simulink model "Position_control_PP"  (R2019b)
settings: Solver=ode1  StartTime=0.0  StopTime=26  FixedStep=0.002  RelTol=1e-3  EnableMultiTasking=on
PostLoadFcn:
  | qc_set_target_type(getConfigSet(bdroot, 'QUARC Default Target Configuration'));
undefined symbols (not defined in the file): __PRM__SERIALIZED__DATA__, HIL, K0pp, K1pp, qc_get_step_size, SubsystemReferenceBlock
libraries: quarc_library x12, SignalEditorBlockLib x9, simulink_extras x7, cstblocks x7, simulink x2
settings Model: SimulationMode=external  ExtModeTrigDuration=10000  Creator=MLevis  LastModifiedBy=Student
settings SolverCC: PositivePriorityOrder=on
settings DataIOCC: LimitDataPoints=on  SaveFormat=Array  SignalLoggingSaveFormat=ModelDataLogs  ReturnWorkspaceOutputs=off
settings OptimizationCC: ExpressionDepthLimit=2147483647  InitFltsAndDblsToZero=on
settings DebuggingCC: SaveWithParameterizedLinksMsg=none  UnderspecifiedInitializationDetection=Classic  MergeDetectMultiDrivingBlocksExec=none  SolverPrmCheckMsg=warning  MultiTaskDSMMsg=warning  MultiTaskCondExecSysMsg=none  FcnCallInpInsideContextMsg=warning  StateNameClashWarn=warning  SFUnexpectedBacktrackingDiag=warning  SFNoUnconditionalDefaultTransitionDiag=warning  SFExecutionAtInitializationDiag=none  ArithmeticOperatorsInVariantConditions=warning
settings HardwareCC: ProdBitPerPointer=32  ProdBitPerSizeT=32  ProdBitPerPtrDiffT=32  ProdLargestAtomicFloat=None  ProdIntDivRoundTo=Undefined  ProdEndianess=Unspecified  ProdWordSize=32  ProdHWDeviceType=32-bit Generic
settings ModelReferenceCC: PropagateSignalLabelsOutOfModel=off
settings SFSimCC: SimUseLocalCustomCode=off  CustomCodeUndefinedFunction=UseInterfaceOnly
settings RTWCC: Description=QUARC Win64 Target  SystemTargetFile=quarc_win64.tlc  TemplateMakefile=quarc_default_tmf  RTWUseLocalCustomCode=off
settings CodeAppCC: StateflowObjectComments=on
settings STFCustomTargetCC: TargetPreCompLibLocation=C:\PROGRA~3\QUARC\lib\2019b\win64\release  ConcurrentExecutionCompliant=on  GRTInterface=on  SystemTargetFile=quarc_win64.tlc
settings GRTTargetCC: TargetPreCompLibLocation=C:\PROGRA~3\QUARC\lib\2019b\win64\release  TargetLangStandard=C89/C90 (ANSI)  ParMdlRefBuildCompliant=off  CompOptLevelCompliant=off  CombineOutputUpdateFcns=off  MatFileLogging=off  CPPClassGenCompliant=off  GRTInterface=on  UseToolchainInfoCompliant=off  ExtMode=on  ExtModeMexFile=quarc_comm
settings ConfigComp: CovMetricSettings=dw  CovHtmlReporting=on  CovSaveCumulativeToWorkspaceVar=on  CovSaveSingleToWorkspaceVar=on  CovExternalEMLEnable=off

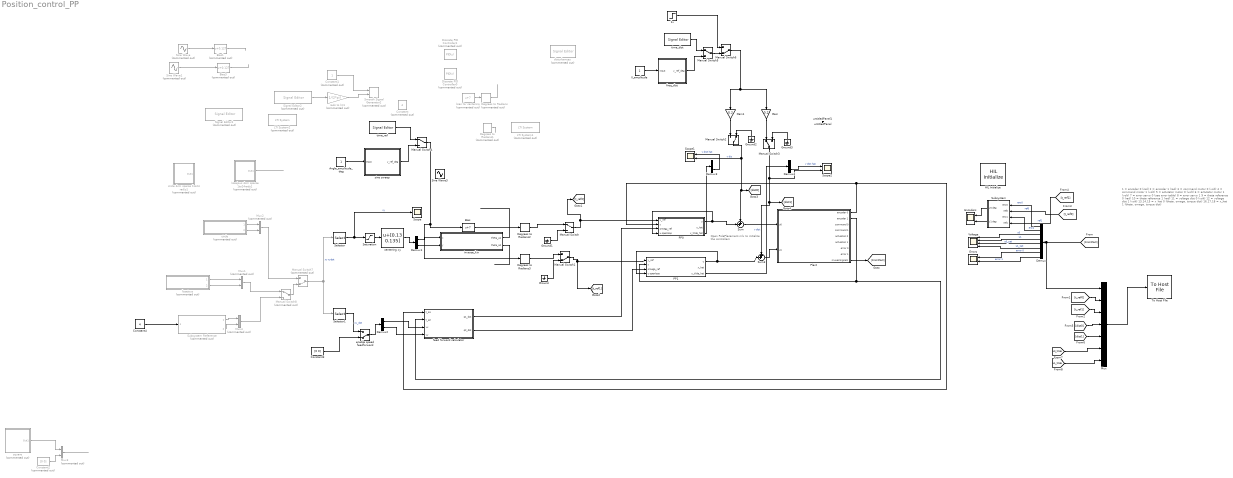
== system Position_control_PP ==
  note: Open PolePlacement.mlx
      | to initialize the controllers
  note: 1 = encoder 0 (rad)
      | 2 = encoder 1 (rad)
      | 3 = command motor 0 (volt)
      | 4 = command motor 1 (volt)
      | 5 = actutator motor 0 (volt)
      | 6 = actutator motor 1 (volt)
      | 7 = error servo 0 (see error table)
      | 8 = error servo 1
      | 9 = theta reference 0 (rad)
      | 10 = theta reference 1 (rad)
      | 11 = voltage dist 0 (volt)
      | 12 = voltage dist 1 (volt)
      | 13,14,15 = x_hat 0 (theta, omega, torque dist)
      | 16,17,18 = x_hat 1 (theta, omega, torque dist)
  1v : Step  SampleTime=0
  Angle_amplitude_deg : Constant
  Bias : Bias  Bias=7
  Bias1 : Bias  Commented=on  Bias=0.127
  Bias3 : Bias  Commented=on  Bias=0.127
  Constant : Constant  Commented=on  Value=4
  Constant1 : Constant  Commented=on
  Constant2 : Constant  Commented=on  Value=[0 0]
  Constant3 : Constant  Value=[0 0]
  Constant4 : Constant  Value=4
  Degrees to Radians : simulink_extras/Transformations/Degrees to Radians  Commented=on
  Degrees to Radians1 : simulink_extras/Transformations/Degrees to Radians  Commented=on
  Degrees to Radians2 : simulink_extras/Transformations/Degrees to Radians
  Degrees to Radians3 : simulink_extras/Transformations/Degrees to Radians
  Demux : Demux  Outputs=8
  Demux1 : Demux  Outputs=2
  Demux2 : Demux  Outputs=2
  Demux3 : Demux  Outputs=3
  Demux4 : Demux  Outputs=3
  Discrete PID Controller0 : simulink/Continuous/PID Controller  Commented=on  Controller=PID  Form=Parallel  TimeDomain=Discrete-time  SampleTime=-1  IntegratorMethod=Forward Euler  FilterMethod=Forward Euler  ControllerParametersSource=internal  P=-21.6  I=0  D=-0.423  UseFilter=on  N=100  TunerSelectOption=Transfer Function Based (PID Tuner App)  InitialConditionSource=internal  InitialConditionForIntegrator=0  InitialConditionForFilter=0  DifferentiatorICPrevScaledInput=0  ExternalReset=none  TrackingMode=off  Kt=1  LimitOutput=off  UpperSaturationLimit=inf  LowerSaturationLimit=-inf  LinearizeAsGain=off  AntiWindupMode=none  Kb=1  POutMin=[]  POutMax=[]  IOutMin=[]  IOutMax=[]  DOutMin=[]  DOutMax=[]  NOutMin=[]  NOutMax=[]  SumOutMin=[]  SumOutMax=[]  SaturationOutMin=[]  SaturationOutMax=[]  PParamMin=[]  PParamMax=[]  IParamMin=[]  IParamMax=[]  DParamMin=[]  DParamMax=[]  NParamMin=[]  NParamMax=[]  KbParamMin=[]  KbParamMax=[]  KtParamMin=[]  KtParamMax=[]  KbOutMin=[]  KbOutMax=[]  KtOutMin=[]  KtOutMax=[]  IntegratorOutMin=[]  IntegratorOutMax=[]  FilterOutMin=[]  FilterOutMax=[]  SumI1OutMin=[]  SumI1OutMax=[]  SumI2OutMin=[]  SumI2OutMax=[]  SumI3OutMin=[]  SumI3OutMax=[]  SumI4OutMin=[]  SumI4OutMax=[]  SumDOutMin=[]  SumDOutMax=[]  DifferentiatorOutMin=[]  DifferentiatorOutMax=[]  FilterDiffOutCoefMin=[]  FilterDiffOutCoefMax=[]  ReciprocalOutMin=[]  ReciprocalOutMax=[]  SumDenOutMin=[]  SumDenOutMax=[]  SumNumOutMin=[]  SumNumOutMax=[]  DivideOutMin=[]  DivideOutMax=[]  IntegratorContinuousStateAttributes=''  IntegratorStateMustResolveToSignalObject=off  IntegratorRTWStateStorageClass=Auto  FilterContinuousStateAttributes=''  FilterStateMustResolveToSignalObject=off  FilterRTWStateStorageClass=Auto  ParallelPVariant=InternalParameters  IdealPVariant=Disabled  IVariant=InternalParameters  DVariant=InternalParameters  IntegratorVariant=Discrete  SatVariant=Disabled  AWVariant=Passthrough  PCopyVariant=Disabled  TRVariant=Disabled  FdbkBlocksVariant=Forward  IdealPFdbkVariant=Disabled  SatFdbkVariant=Disabled  DerivativeFilterVariant=ForwardEulerFilter  NVariant=InternalParameters  NCopyVariant=Disabled  FilterICVariant=InternalICsFilter  IntegratorICVariant=InternalICs  ExternalResetVariant=Disabled  TRSumVariant=Passthrough  SumFdbkVariant=Disabled  SumVariant=Sum_PID
  Discrete PID Controller1 : simulink/Continuous/PID Controller  Commented=on  Controller=PID  Form=Parallel  TimeDomain=Discrete-time  SampleTime=-1  IntegratorMethod=Forward Euler  FilterMethod=Forward Euler  ControllerParametersSource=internal  P=-21.4  I=0  D=-0.43  UseFilter=on  N=100  TunerSelectOption=Transfer Function Based (PID Tuner App)  InitialConditionSource=internal  InitialConditionForIntegrator=0  InitialConditionForFilter=0  DifferentiatorICPrevScaledInput=0  ExternalReset=none  TrackingMode=off  Kt=1  LimitOutput=off  UpperSaturationLimit=inf  LowerSaturationLimit=-inf  LinearizeAsGain=off  AntiWindupMode=none  Kb=1  POutMin=[]  POutMax=[]  IOutMin=[]  IOutMax=[]  DOutMin=[]  DOutMax=[]  NOutMin=[]  NOutMax=[]  SumOutMin=[]  SumOutMax=[]  SaturationOutMin=[]  SaturationOutMax=[]  PParamMin=[]  PParamMax=[]  IParamMin=[]  IParamMax=[]  DParamMin=[]  DParamMax=[]  NParamMin=[]  NParamMax=[]  KbParamMin=[]  KbParamMax=[]  KtParamMin=[]  KtParamMax=[]  KbOutMin=[]  KbOutMax=[]  KtOutMin=[]  KtOutMax=[]  IntegratorOutMin=[]  IntegratorOutMax=[]  FilterOutMin=[]  FilterOutMax=[]  SumI1OutMin=[]  SumI1OutMax=[]  SumI2OutMin=[]  SumI2OutMax=[]  SumI3OutMin=[]  SumI3OutMax=[]  SumI4OutMin=[]  SumI4OutMax=[]  SumDOutMin=[]  SumDOutMax=[]  DifferentiatorOutMin=[]  DifferentiatorOutMax=[]  FilterDiffOutCoefMin=[]  FilterDiffOutCoefMax=[]  ReciprocalOutMin=[]  ReciprocalOutMax=[]  SumDenOutMin=[]  SumDenOutMax=[]  SumNumOutMin=[]  SumNumOutMax=[]  DivideOutMin=[]  DivideOutMax=[]  IntegratorContinuousStateAttributes=''  IntegratorStateMustResolveToSignalObject=off  IntegratorRTWStateStorageClass=Auto  FilterContinuousStateAttributes=''  FilterStateMustResolveToSignalObject=off  FilterRTWStateStorageClass=Auto  ParallelPVariant=InternalParameters  IdealPVariant=Disabled  IVariant=InternalParameters  DVariant=InternalParameters  IntegratorVariant=Discrete  SatVariant=Disabled  AWVariant=Passthrough  PCopyVariant=Disabled  TRVariant=Disabled  FdbkBlocksVariant=Forward  IdealPFdbkVariant=Disabled  SatFdbkVariant=Disabled  DerivativeFilterVariant=ForwardEulerFilter  NVariant=InternalParameters  NCopyVariant=Disabled  FilterICVariant=InternalICsFilter  IntegratorICVariant=InternalICs  ExternalResetVariant=Disabled  TRSumVariant=Passthrough  SumFdbkVariant=Disabled  SumVariant=Sum_PID
  Encoders : Scope  NumInputPorts=2
  Errors : Scope  NumInputPorts=2
  Gain : Gain  Gain=0.2
  Gain1 : Gain  Gain=0.2
  Ground{,1..3} (4 alike) : Ground
  HIL Initialize : quarc_library/Data Acquisition/Generic/Configuration/HIL Initialize  object_name=HIL-1  board_type=q2_usb  board_number=0  board_options=d0=digital;d1=digital;led=auto;update_rate=normal;decimation=1  exclusive=off  active=off  hardware_clocks=[0]  clock_modes=[]  initial_clock_frequencies=[]  set_clock_params_at_start=off  set_clock_params_at_switch_in=off  set_clock_frequencies_at_start=off  set_clock_frequencies_at_switch_in=off  analog_input_channels=[0:1]  analog_input_configurations=[]  analog_input_maximums=10  analog_input_minimums=-10  set_analog_input_params_at_start=on  set_analog_input_params_at_switch_in=off  analog_output_channels=[0:1]  analog_output_maximums=10  analog_output_minimums=-10  initial_analog_outputs=[0]  final_analog_outputs=[0]  watchdog_analog_outputs=0  set_analog_output_params_at_start=on  set_analog_output_params_at_switch_in=off  set_analog_outputs_at_start=on  set_analog_outputs_at_switch_in=off  set_analog_outputs_at_terminate=on  set_analog_outputs_at_switch_out=off  set_analog_outputs_on_watchdog=off  digital_input_channels=[]  digital_output_channels=[]  digital_output_configuration=[]  initial_digital_outputs=[1]  final_digital_outputs=[1]  watchdog_digital_outputs=[1]  set_digital_output_params_at_start=off  set_digital_output_params_at_switch_in=off  set_digital_outputs_at_start=on  set_digital_outputs_at_switch_in=off  set_digital_outputs_at_terminate=on  set_digital_outputs_at_switch_out=off  set_digital_outputs_on_watchdog=off  encoder_channels=[0:1]  quadrature=[4]  encoder_filter_frequency=[]  initial_encoder_counts=[0]  set_encoder_params_at_start=on  set_encoder_params_at_switch_in=off  set_encoder_counts_at_start=on  set_encoder_counts_at_switch_in=off  pwm_channels=[]  pwm_modes=[0]  pwm_frequency=1/0.020  pwm_configuration=[]  pwm_alignment=[]  pwm_polarity=[]  pwm_leading_deadband=[]  pwm_trailing_deadband=[]  initial_pwm_outputs=[0]  final_pwm_outputs=[0]  watchdog_pwm_outputs=[0]  set_pwm_params_at_start=on  set_pwm_params_at_switch_in=off  set_pwm_outputs_at_start=on  set_pwm_outputs_at_switch_in=off  set_pwm_outputs_at_terminate=on  set_pwm_outputs_at_switch_out=off  set_pwm_outputs_on_watchdog=off  other_output_channels=[]  initial_other_outputs=[]  final_other_outputs=[]  watchdog_other_outputs=[]  set_other_outputs_at_start=off  set_other_outputs_at_switch_in=off  set_other_outputs_at_terminate=off  set_other_outputs_at_switch_out=off  set_other_outputs_on_watchdog=off
  LTI System1 : cstblocks/LTI System  Commented=on  sys=C1  IC=[]
  LTI System2 : cstblocks/LTI System  Commented=on  sys=C0  IC=[]
  Manual Switch{,3..5} (4 alike) : ManualSwitch
  Manual Switch1 : ManualSwitch  CurrentSetting=0
  Manual Switch2 : ManualSwitch  CurrentSetting=0
  Manual Switch6 : ManualSwitch  CurrentSetting=0
  Manual Switch7 : ManualSwitch  Commented=on  CurrentSetting=0
  Manual Switch8 : ManualSwitch  Commented=on
  Mux : Mux  Inputs=7
  Mux{1..4} (4 alike) : Mux  Commented=on  Inputs=2
  PP0 : Subsystem
  PP1 : Subsystem
  Plant : Subsystem  mask(Plant with checks){LowSat=10.0, HighSat=0.330, A0min=-17, A0max=31, A0slack=1, bias=off, A1min=-27, A1max=27, A1slack=1}
      mask prompts: LowSat "Nominal Saturation"; HighSat "Safety Saturation"; A0min "A1 Min"; A0max "A1 Max"; A0slack "A1 Slack"; bias "Use cartesian reference"; A1min "A2 Min"; A1max "A2 Max"; A1slack "A2 Slack"
      mask help: All angles described in DEGREES with respect to the markings on the physical system (unless the toggle is checked)
      mask DialogControl Container9 Prompt: Voltages
      mask DialogControl Container9_copy Prompt: Angle Limits
      mask DialogControl ParameterGroupVar Prompt: Theta A1 (Motor 0)
      mask DialogControl Container8 Prompt: Theta A2 (Motor 1)
      mask DialogControl Control2 Prompt: When enabled uses the canonical angles instead of the displacement from resting position
      mask Display: image('$imagefile'); % Use "Edit Image" on toolstrip to change.
  Saturation : Saturate  UpperLimit=0.04  LowerLimit=-0.04
  Scope : Scope
  Scope1 : Scope  NumInputPorts=2
  Scope2 : Scope  NumInputPorts=2
  Selector : Selector  InputPortWidth=4  IndexOptions=Index vector (dialog)  Indices=[1 2]  OutputSizes=1
  Selector1 : Selector  InputPortWidth=4  IndexOptions=Index vector (dialog)  Indices=[3 4]  OutputSizes=1
  Signal Editor1 : SignalEditorBlockLib/Signal Editor  Commented=on  FileName=D:\Users\icpmoles\my\polimi\università\Magistrale 2 anno 2 semestre\lab\ASB\lab5\preplan\stairs.mat  ActiveScenario=x1to35sparse  ActiveSignal=Signal  IsBus=off  OutputBusObjectStr=Bus: BusObject  SampleTime=0  Interpolate=off  ZeroCross=off  OutputAfterFinalValue=Setting to zero  Unit=inherit  PreserveSignalName=on
      settings: SourceProductName=Simulink
  Signal Editor2 : SignalEditorBlockLib/Signal Editor  Commented=on  FileName=C:\Users\Student\Downloads\CNC (4)\CNC\sinesweep\lab4\stairs.mat  ActiveScenario=x1to30with10s_pause  ActiveSignal=Signal 1  IsBus=off  OutputBusObjectStr=Bus: BusObject  SampleTime=0  Interpolate=off  ZeroCross=off  OutputAfterFinalValue=Holding final value  Unit=inherit  PreserveSignalName=on
      settings: SourceProductName=Simulink
  Sine Wave : Sin  Commented=on  Amplitude=0.03  Frequency=2  Phase=pi/2  SampleTime=0
  Sine Wave1 : Sin  Commented=on  Amplitude=0.03  Frequency=2  SampleTime=0
  Sine Wave3 : Sin  Amplitude=0.5  Frequency=5  SampleTime=0
  Smooth Signal Generator2 : quarc_library/Sources/Signals/Smooth Signal Generator  Commented=on  signal_type=Sine  source=External (input ports)  amplitude=1  frequency=1  initial_phase=0  sample_time=qc_get_step_size  output_cos=off
      settings: SourceProductName=QUARC Targets
  Subsystem : Subsystem
  Subsystem Reference : Subsystem  Commented=on  BlockKeywords=__PRM__SERIALIZED__DATA__:SubsystemReferenceBlock  ReferencedSubsystem=square_generator
  Sum : Sum  Inputs=++|
  Sum3 : Sum  Inputs=++|
  To Host File : quarc_library/Sinks/To Host/To Host File  file_name=%m_%{date}_%{time}.mat  variable_name=data  decimation=1  sample_time=-1  file_format=MAT-file v.4  options=No header or footer  append=off  final_file_name=Position_control_PP_29-Apr-2025_18-49-00.mat  bitrate=2000000
  V_amplitude : Constant
  Voltage : Scope  NumInputPorts=4
  bias for centering : Bias  Commented=on  Bias=7
  centering xy : Bias  Bias=[0.13 0.135]
  circle : Subsystem  Commented=on  BlockKeywords=__PRM__SERIALIZED__DATA__:SubsystemReferenceBlock  ReferencedSubsystem=circle_generator
  circle 4cm sparse 1to24 rad/s1 : Subsystem  Commented=on
  disturbances : SignalEditorBlockLib/Signal Editor  Commented=on  FileName=D:\Users\icpmoles\my\polimi\università\Magistrale 2 anno 2 semestre\lab\ASB\lab5\preplan\scenario.mat  ActiveScenario=WhiteNoise  ActiveSignal=m0  IsBus=off  OutputBusObjectStr=Bus: BusObject  SampleTime=0  Interpolate=off  ZeroCross=off  OutputAfterFinalValue=Setting to zero  Unit=V  PreserveSignalName=on
      settings: SourceProductName=Simulink
  enable speed feedforward : ManualSwitch  CurrentSetting=0
  feed forward calculator : MATLAB Function  TreatAsAtomicUnit=on
  freq_dist : Subsystem
  "inverse_kin " : Subsystem
  lissajous : Subsystem  Commented=on  BlockKeywords=__PRM__SERIALIZED__DATA__:SubsystemReferenceBlock  ReferencedSubsystem=lissajous_generator
  lissajous 4cm sparse 1to24rads1 : Subsystem  Commented=on
  rads to hz1 : Gain  Commented=on  Gain=1/(2*pi)
  sine sweep : Subsystem
  square : Subsystem  Commented=on
  time_dist : SignalEditorBlockLib/Signal Editor  FileName=angle_ref_scenario_time.mat  ActiveScenario=whitenoise_5to1  ActiveSignal=Signal  IsBus=off  OutputBusObjectStr=Bus: BusObject  SampleTime=0  Interpolate=off  ZeroCross=off  OutputAfterFinalValue=Setting to zero  Unit=inherit  PreserveSignalName=on
      settings: SourceProductName=Simulink
  time_ref : SignalEditorBlockLib/Signal Editor  FileName=angle_ref_scenario_time.mat  ActiveScenario=square_dyn_15to5  ActiveSignal=Signal  IsBus=off  OutputBusObjectStr=Bus: BusObject  SampleTime=0  Interpolate=off  ZeroCross=off  OutputAfterFinalValue=Setting to zero  Unit=inherit  PreserveSignalName=on
      settings: SourceProductName=Simulink
  untitledPanel : Subsystem  Tag=HiddenForWebPanel  IsWebBlockPanel=on
  untitledPanel1 : Subsystem  Tag=HiddenForWebPanel  IsWebBlockPanel=on
  wires:
  Plant/1(encoder 0) -> PP0/2(y), feed forward calculator/1(t_a1)
  Plant/2(encoder 1) -> PP1/2(y), feed forward calculator/2(t_a2)
  PP0/1(u) -> PP0/4(u openloop), Sum/2
  Plant/9(muxed signals) -> [FromPlant]
  [FromPlant] -> Mux/1, Demux/1
  Demux/2 -> Subsystem/3(enc1)  "enc1"
  Demux/3 -> Voltage/1  "u0"
  Demux/4 -> Voltage/2  "u1"
  Demux/5 -> Voltage/3  "u0_sat"
  Demux/6 -> Voltage/4  "u1_sat"
  Demux/7 -> Errors/1  "error 0"
  Demux/8 -> Errors/2  "error 1"
  Manual Switch1/1 -> PP1/1(y_ref), [t_ref1]
  Sum/1 -> Plant/1(u0)
  PP1/1(u) -> PP1/4(u openloop), Sum3/2
  Sum3/1 -> Plant/2(u1)
  Mux/1 -> To Host File/1
  Manual Switch/1 -> [t_ref0], PP0/1(y_ref)
  [t_ref0] -> Mux/2
  [t_ref1] -> Mux/3
  Degrees to Radians/1 -> ?
  Degrees to Radians1/1 -> ?
  Ground/1 -> Manual Switch1/2
  Ground1/1 -> Manual Switch/2
  Manual Switch2/1 -> [dist0], Sum/1, Scope1/2  "v dis"
  Ground2/1 -> Manual Switch2/2
  bias for centering/1 -> Degrees to Radians/1
  Gain/1 -> Manual Switch3/1
  Gain1/1 -> Manual Switch2/1
  [dist0] -> Mux/4
  [dist1] -> Mux/5
  rads to hz1/1 -> Smooth Signal Generator2/2
  Constant1/1 -> Smooth Signal Generator2/1
  Signal Editor2/1 -> rads to hz1/1
  Bias1/1 -> ?
  Bias3/1 -> ?
  Sine Wave/1 -> Bias1/1
  Sine Wave1/1 -> Bias3/1
  Ground3/1 -> Manual Switch3/2
  [t_ref0] -> Subsystem/2(ref0)  "ref0"
  Demux/1 -> Subsystem/1(enc0)  "enc0"
  [t_ref1] -> Subsystem/4(ref1)  "ref1"
  Subsystem/1(y0 deg) -> Encoders/1
  Subsystem/2(y1 deg) -> Encoders/2
  ? -> Degrees to Radians1/1, bias for centering/1
  time_ref/1 -> Manual Switch4/1
  time_dist/1 -> Manual Switch5/1
  freq_dist/1(y_ref_deg) -> Manual Switch5/2
  Manual Switch6/1 -> Gain/1, Gain1/1
  V_amplitude/1 -> freq_dist/1(Input)
  Angle_amplitude_deg/1 -> sine sweep/1(Input)
  [x0_tilde] -> Mux/6
  [x1_tilde] -> Mux/7
  Manual Switch4/1 -> Bias/1, Degrees to Radians3/1
  lissajous 4cm sparse 1to24rads1/1(Out1) -> ?
  Mux2/1 -> Manual Switch7/1
  Manual Switch7/1 -> Selector1/1, Selector/1  "xy xydot"
  Demux1/1 -> "inverse_kin "/1(x)
  Demux1/2 -> "inverse_kin "/2(y)
  "inverse_kin "/1(theta_a1) -> ?
  "inverse_kin "/2(theta_a2) -> ?
  Manual Switch8/1 -> Manual Switch7/2
  square/1(Out1) -> Mux3/1
  Manual Switch5/1 -> Manual Switch6/2
  1v/1 -> Manual Switch6/1
  Mux1/1 -> Manual Switch8/1
  lissajous/1 -> Mux1/1
  lissajous/2 -> Mux1/2
  circle/1 -> Mux2/1
  circle/2 -> Mux2/2
  Selector/1 -> Scope/1, Saturation/1  "xy"
  Mux3/1 -> ?
  Constant2/1 -> Mux3/2
  Selector1/1 -> enable speed feedforward/1  "xy_dot"
  Demux2/1 -> feed forward calculator/3(vx)
  Demux2/2 -> feed forward calculator/4(vy)
  feed forward calculator/1(q1_dot) -> PP0/3(omega_ref)
  enable speed feedforward/1 -> Demux2/1
  Constant3/1 -> enable speed feedforward/2
  feed forward calculator/2(q2_dot) -> PP1/3(omega_ref)
  Subsystem Reference/1 -> Mux4/1
  Subsystem Reference/2 -> Mux4/2
  Constant4/1 -> Subsystem Reference/1
  Mux4/1 -> Manual Switch8/2
  centering xy/1 -> Demux1/1
  Saturation/1 -> centering xy/1
  PP0/3(x_tilde_hat) -> Demux3/1
  Demux3/3 -> Scope1/1  "v dist hat"
  PP1/3(x_tilde_hat) -> Demux4/1
  Demux4/3 -> Scope2/1  "v dist hat"
  Manual Switch3/1 -> Scope2/2, Sum3/1, [dist1]  "v dist"
  sine sweep/1(y_ref_deg) -> Manual Switch4/2
  Bias/1 -> Degrees to Radians2/1
  Degrees to Radians2/1 -> Manual Switch/1
  Degrees to Radians3/1 -> Manual Switch1/1

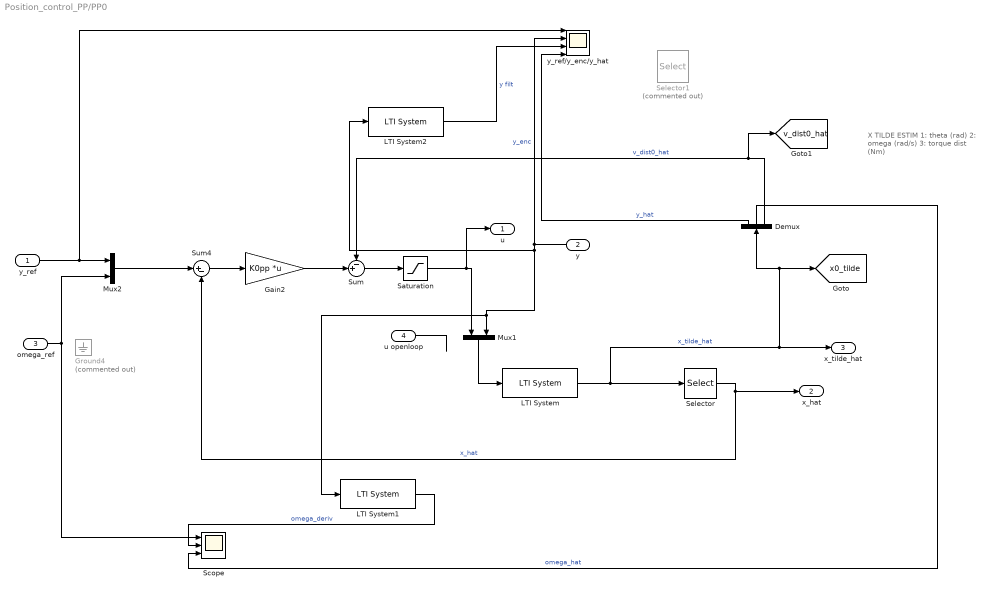
== system Position_control_PP/PP0 ==
  note: X TILDE ESTIM
      | 1: theta (rad)
      | 2: omega (rad/s)
      | 3: torque dist (Nm)
  y_ref : Inport
  y : Inport  Port=2
  omega_ref : Inport  Port=3
  u openloop : Inport  Port=4
  Demux : Demux  Outputs=3
  Gain2 : Gain  Gain=K0pp  Multiplication=Matrix(K*u)
  Ground4 : Ground  Commented=on
  LTI System : cstblocks/LTI System  sys=sysObserver0t  IC=[]
  LTI System1 : cstblocks/LTI System  sys=tf([1 0],[1/20 1])  IC=[]
  LTI System2 : cstblocks/LTI System  sys=tf([1],[1/20 1])  IC=[]
  Mux1 : Mux  Inputs=2
  Mux2 : Mux  Inputs=2
  Saturation : Saturate  UpperLimit=10  LowerLimit=-10
  Scope : Scope  NumInputPorts=3
  Selector : Selector  InputPortWidth=3  IndexOptions=Index vector (dialog)  Indices=[1 2]  OutputSizes=1
  Selector1 : Selector  Commented=on  InputPortWidth=3  IndexOptions=Index vector (dialog)  Indices=3  OutputSizes=1
  Sum : Sum  Inputs=-+|
  Sum4 : Sum  Inputs=|+-
  y_ref/y_enc/y_hat : Scope  NumInputPorts=4
  u : Outport
  x_hat : Outport  Port=2
  x_tilde_hat : Outport  Port=3
  tag scope: v_dist0_hat=global, x0_tilde=global
  wires:
  Selector/1 -> x_hat/1, Sum4/2  "x_hat"
  Sum4/1 -> Gain2/1
  Gain2/1 -> Sum/2
  Mux1/1 -> LTI System/1
  omega_ref/1 -> Mux2/2, Scope/1
  Mux2/1 -> Sum4/1
  Saturation/1 -> Mux1/1, u/1
  LTI System/1 -> Selector/1, Demux/1, [x0_tilde], x_tilde_hat/1  "x_tilde_hat"
  y/1 -> y_ref/y_enc/y_hat/2, LTI System1/1, Mux1/2, LTI System2/1  "y_enc"
  y_ref/1 -> y_ref/y_enc/y_hat/1, Mux2/1
  Sum/1 -> Saturation/1
  Demux/3 -> [v_dist0_hat], Sum/1  "v_dist0_hat"
  Demux/1 -> y_ref/y_enc/y_hat/4  "y_hat"
  Demux/2 -> Scope/3  "omega_hat"
  LTI System1/1 -> Scope/2  "omega_deriv"
  LTI System2/1 -> y_ref/y_enc/y_hat/3  "y filt"
  u openloop/1 -> ?

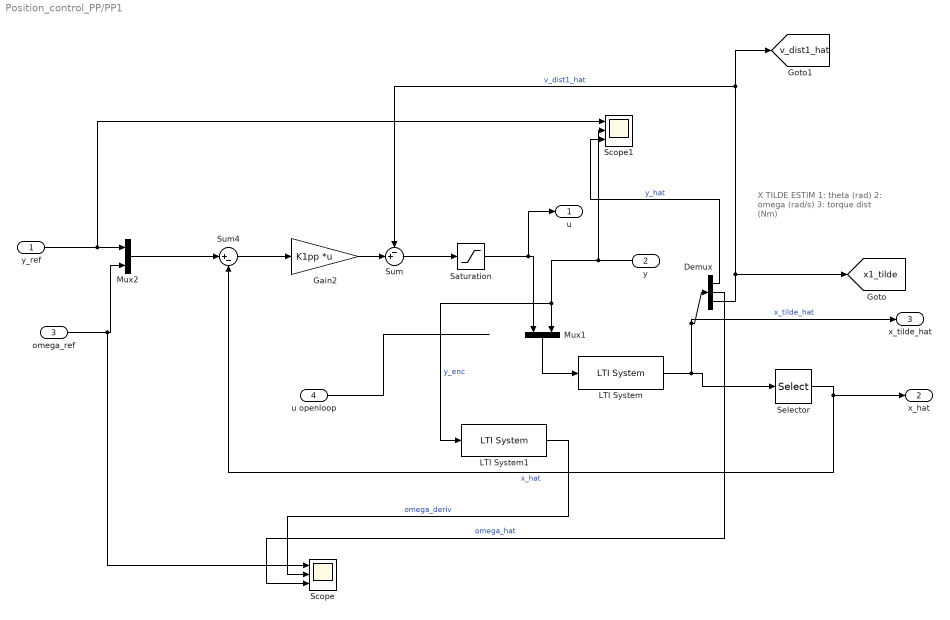
== system Position_control_PP/PP1 ==
  note: X TILDE ESTIM
      | 1: theta (rad)
      | 2: omega (rad/s)
      | 3: torque dist (Nm)
  y_ref : Inport
  y : Inport  Port=2
  omega_ref : Inport  Port=3
  u openloop : Inport  Port=4
  Demux : Demux  Outputs=3
  Gain2 : Gain  Gain=K1pp  Multiplication=Matrix(K*u)
  LTI System : cstblocks/LTI System  sys=sysObserver1t  IC=[]
  LTI System1 : cstblocks/LTI System  sys=tf([1 0],[1/20 1])  IC=[]
  Mux1 : Mux  Inputs=2
  Mux2 : Mux  Inputs=2
  Saturation : Saturate  UpperLimit=10  LowerLimit=-10
  Scope : Scope  NumInputPorts=3
  Scope1 : Scope  NumInputPorts=3
  Selector : Selector  InputPortWidth=3  IndexOptions=Index vector (dialog)  Indices=[1 2]  OutputSizes=1
  Sum : Sum  Inputs=-+|
  Sum4 : Sum  Inputs=|+-
  u : Outport
  x_hat : Outport  Port=2
  x_tilde_hat : Outport  Port=3
  tag scope: v_dist1_hat=global, x1_tilde=global
  wires:
  Selector/1 -> x_hat/1, Sum4/2  "x_hat"
  Sum4/1 -> Gain2/1
  Gain2/1 -> Sum/2
  Mux1/1 -> LTI System/1
  omega_ref/1 -> Scope/1, Mux2/2
  Mux2/1 -> Sum4/1
  Saturation/1 -> Mux1/1, u/1
  LTI System/1 -> x_tilde_hat/1, Demux/1, Selector/1  "x_tilde_hat"
  y_ref/1 -> Scope1/1, Mux2/1
  Demux/3 -> [v_dist1_hat], Sum/1, [x1_tilde]  "v_dist1_hat"
  Sum/1 -> Saturation/1
  LTI System1/1 -> Scope/2  "omega_deriv"
  Demux/2 -> Scope/3  "omega_hat"
  y/1 -> Scope1/2, LTI System1/1, Mux1/2  "y_enc"
  Demux/1 -> Scope1/3  "y_hat"
  u openloop/1 -> ?

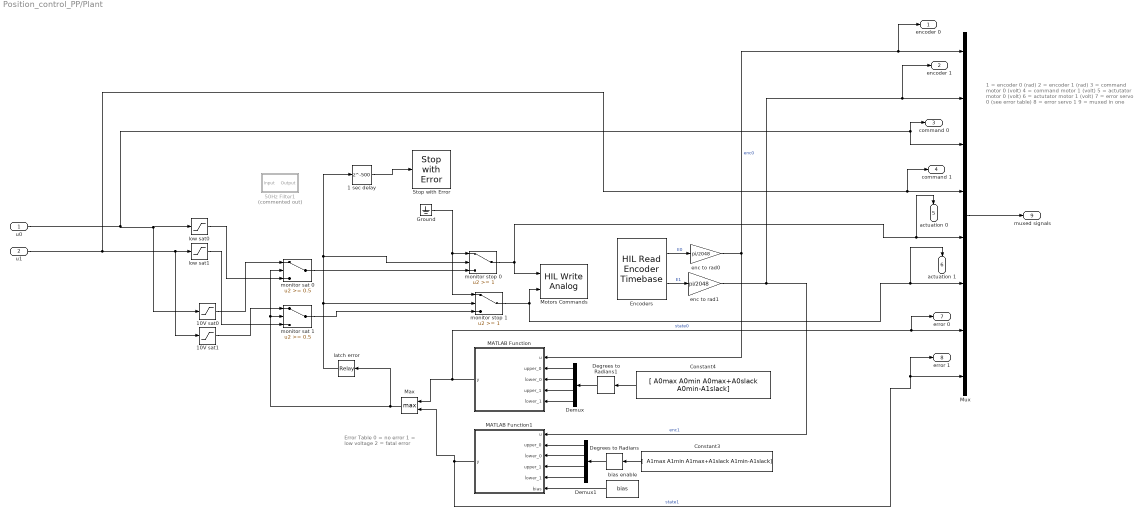
== system Position_control_PP/Plant ==
  note: Error Table
      | 0 = no error
      | 1 = low voltage
      | 2 = fatal error
  note: 1 = encoder 0 (rad)
      | 2 = encoder 1 (rad)
      | 3 = command motor 0 (volt)
      | 4 = command motor 1 (volt)
      | 5 = actutator motor 0 (volt)
      | 6 = actutator motor 1 (volt)
      | 7 = error servo 0 (see error table)
      | 8 = error servo 1
      | 9 = muxed in one
  u0 : Inport  Unit=V
  u1 : Inport  Port=2  Unit=V
  1 sec delay : Delay  DelayLength=500
  10V sat0 : Saturate  UpperLimit=HighSat  LowerLimit=-HighSat
  10V sat1 : Saturate  UpperLimit=HighSat  LowerLimit=-HighSat
  50Hz Filter1 : Subsystem  Tag=FilterWizardSubSystem  Commented=on
      settings: ErrorFcn=dspFilterRealizedInBasicElemsAlgLoopErrFcnCallback
  Constant3 : Constant  Value="[  A1max A1min A1max+A1slack A1min-A1slack]"
  Constant4 : Constant  Value="[  A0max A0min A0max+A0slack A0min-A1slack]"
  Degrees to Radians : simulink_extras/Transformations/Degrees to Radians
  Degrees to Radians1 : simulink_extras/Transformations/Degrees to Radians
  Demux : Demux
  Demux1 : Demux
  Encoders : quarc_library/Data Acquisition/Generic/Timebases/HIL Read Encoder Timebase  object_name=HIL-1  clock=0  channels=0:1  samples_in_buffer=max(ceil(1/qc_get_step_size), 1)  active=on  vector_output=off  data_type_mode=Inherit via back propagation  data_type=double
  Ground : Ground
  MATLAB Function : MATLAB Function  TreatAsAtomicUnit=on
  MATLAB Function1 : MATLAB Function  TreatAsAtomicUnit=on
  Max : MinMax  Function=max  Inputs=2
  Motors Commands : quarc_library/Data Acquisition/Generic/Immediate I//O/HIL Write Analog  object_name=HIL-1  channels=0:1  sample_time=-1  active=off  vector_input=off
  Mux : Mux  Inputs=8
  Stop with Error : quarc_library/Sinks/Error Handling/Stop with Error  message_type=Fixed error message  message=Out of bounds
      settings: AttributesFormatString="\"%<message>\""  SourceProductName=QUARC Targets
  bias enable : Constant  Value=bias
  enc to rad0 : Gain  Gain=pi/2048
  enc to rad1 : Gain  Gain=pi/2048
  latch error : Relay  OnSwitchValue=2  OffSwitchValue=-1
  low sat0 : Saturate  UpperLimit=LowSat  LowerLimit=-LowSat
  low sat1 : Saturate  UpperLimit=LowSat  LowerLimit=-LowSat
  monitor sat 0 : Switch  Threshold=0.5
  "monitor sat 1 " : Switch  Threshold=0.5
  monitor stop 0 : Switch  Threshold=1
  monitor stop 1 : Switch  Threshold=1
  encoder 0 : Outport  Unit=rad
  encoder 1 : Outport  Port=2  Unit=rad
  command 0 : Outport  Port=3  Unit=V
  command 1 : Outport  Port=4  Unit=V
  actuation 0 : Outport  Port=5  Unit=V
  actuation 1 : Outport  Port=6  Unit=V
  error 0 : Outport  Port=7
  error 1 : Outport  Port=8
  muxed signals : Outport  Port=9
  wires:
  MATLAB Function1/1(y) -> Max/2, error 1/1, Mux/8  "state1"
  Max/1 -> monitor sat 0/2, "monitor sat 1 "/2, latch error/1
  enc to rad1/1 -> encoder 1/1, Mux/2, MATLAB Function1/1(u)  "enc1"
  latch error/1 -> monitor stop 1/2, monitor stop 0/2, 1 sec delay/1
  low sat0/1 -> monitor sat 0/3
  monitor stop 1/1 -> Motors Commands/2, actuation 1/1, Mux/6
  u0/1 -> low sat0/1, 10V sat0/1, command 0/1, Mux/3
  10V sat1/1 -> "monitor sat 1 "/1
  Demux1/2 -> MATLAB Function1/3(lower_0)
  enc to rad0/1 -> MATLAB Function/1(u), encoder 0/1, Mux/1  "enc0"
  Demux1/4 -> MATLAB Function1/5(lower_1)
  low sat1/1 -> "monitor sat 1 "/3
  Demux1/1 -> MATLAB Function1/2(upper_0)
  Encoders/2 -> enc to rad1/1  "E1"
  Demux/1 -> MATLAB Function/2(upper_0)
  MATLAB Function/1(y) -> error 0/1, Mux/7, Max/1  "state0"
  Demux1/3 -> MATLAB Function1/4(upper_1)
  u1/1 -> 10V sat1/1, low sat1/1, command 1/1, Mux/4
  Demux/4 -> MATLAB Function/5(lower_1)
  Demux/3 -> MATLAB Function/4(upper_1)
  Demux/2 -> MATLAB Function/3(lower_0)
  Encoders/1 -> enc to rad0/1  "E0"
  Mux/1 -> muxed signals/1
  1 sec delay/1 -> Stop with Error/1
  10V sat0/1 -> monitor sat 0/1
  Constant3/1 -> Degrees to Radians/1
  Degrees to Radians/1 -> Demux1/1
  Constant4/1 -> Degrees to Radians1/1
  Degrees to Radians1/1 -> Demux/1
  bias enable/1 -> MATLAB Function1/6(bias)
  monitor stop 0/1 -> actuation 0/1, Mux/5, Motors Commands/1
  "monitor sat 1 "/1 -> monitor stop 1/3
  Ground/1 -> monitor stop 1/1, monitor stop 0/1
  monitor sat 0/1 -> monitor stop 0/3

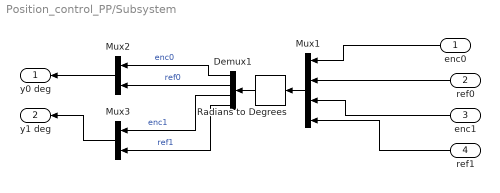
== system Position_control_PP/Subsystem ==
  enc0 : Inport
  ref0 : Inport  Port=2
  enc1 : Inport  Port=3
  ref1 : Inport  Port=4
  Demux1 : Demux
  Mux1 : Mux
  Mux2 : Mux  Inputs=2
  Mux3 : Mux  Inputs=2
  Radians to Degrees : simulink_extras/Transformations/Radians to Degrees
  y0 deg : Outport
  y1 deg : Outport  Port=2
  wires:
  Demux1/1 -> Mux2/1  "enc0"
  Radians to Degrees/1 -> Demux1/1
  Demux1/3 -> Mux3/1  "enc1"
  enc1/1 -> Mux1/3
  Demux1/2 -> Mux2/2  "ref0"
  ref0/1 -> Mux1/2
  Mux1/1 -> Radians to Degrees/1
  Demux1/4 -> Mux3/2  "ref1"
  enc0/1 -> Mux1/1
  ref1/1 -> Mux1/4
  Mux3/1 -> y1 deg/1
  Mux2/1 -> y0 deg/1

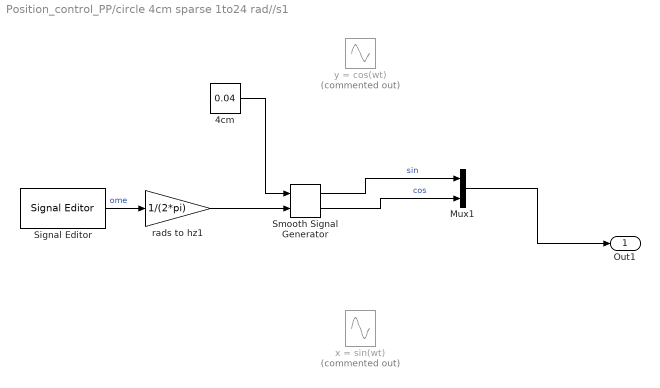
== system Position_control_PP/circle 4cm sparse 1to24 rad//s1 ==
  4cm : Constant  Value=0.04
  Mux1 : Mux  Inputs=2
  Signal Editor : SignalEditorBlockLib/Signal Editor  FileName=circle_omega.mat  ActiveScenario=circle  ActiveSignal=wxy  IsBus=off  OutputBusObjectStr=Bus: BusObject  SampleTime=0  Interpolate=off  ZeroCross=off  OutputAfterFinalValue=Setting to zero  Unit=inherit  PreserveSignalName=on
      settings: SourceProductName=Simulink
  Smooth Signal Generator : quarc_library/Sources/Signals/Smooth Signal Generator  signal_type=Sine  source=External (input ports)  amplitude=1  frequency=1  initial_phase=0  sample_time=qc_get_step_size  output_cos=on
      settings: SourceProductName=QUARC Targets
  rads to hz1 : Gain  Gain=1/(2*pi)
  x = sin(wt) : Sin  Commented=on  Amplitude=0.04  Frequency=2  SampleTime=0
  y = cos(wt) : Sin  Commented=on  Amplitude=0.04  Frequency=2  Phase=pi/2  SampleTime=0
  Out1 : Outport
  wires:
  Smooth Signal Generator/1 -> Mux1/1  "sin"
  Smooth Signal Generator/2 -> Mux1/2  "cos"
  Mux1/1 -> Out1/1
  Signal Editor/1 -> rads to hz1/1  "ome"
  rads to hz1/1 -> Smooth Signal Generator/2
  4cm/1 -> Smooth Signal Generator/1

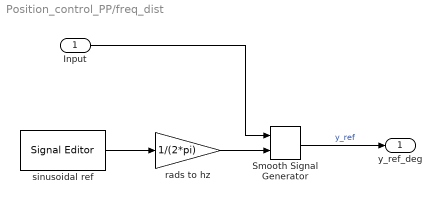
== system Position_control_PP/freq_dist ==
  Input : Inport
  Smooth Signal Generator : quarc_library/Sources/Signals/Smooth Signal Generator  signal_type=Sine  source=External (input ports)  amplitude=1  frequency=1  initial_phase=0  sample_time=qc_get_step_size  output_cos=off
      settings: SourceProductName=QUARC Targets
  rads to hz : Gain  Gain=1/(2*pi)
  sinusoidal ref : SignalEditorBlockLib/Signal Editor  FileName=angle_ref_scenario_freq.mat  ActiveScenario=x1to34_sparse  ActiveSignal=Signal 1  IsBus=off  OutputBusObjectStr=Bus: BusObject  SampleTime=0  Interpolate=off  ZeroCross=off  OutputAfterFinalValue=Holding final value  Unit=inherit  PreserveSignalName=on
      settings: SourceProductName=Simulink
  y_ref_deg : Outport
  wires:
  sinusoidal ref/1 -> rads to hz/1
  rads to hz/1 -> Smooth Signal Generator/2
  Smooth Signal Generator/1 -> y_ref_deg/1  "y_ref"
  Input/1 -> Smooth Signal Generator/1

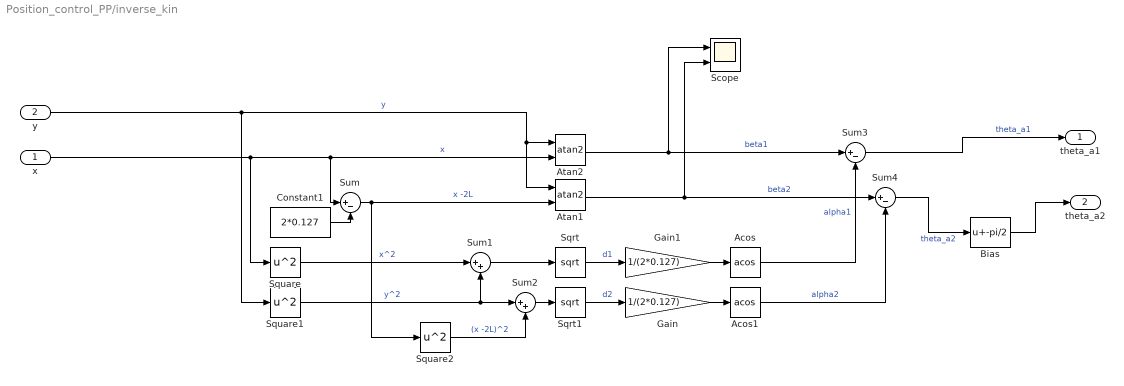
== system Position_control_PP/inverse_kin  ==
  x : Inport
  y : Inport  Port=2
  Acos : Trigonometry  Operator=acos
  Acos1 : Trigonometry  Operator=acos
  Atan1 : Trigonometry  Operator=atan2
  Atan2 : Trigonometry  Operator=atan2
  Bias : Bias  Bias=-pi/2
  Constant1 : Constant  Value=2*0.127
  Gain : Gain  Gain=1/(2*0.127)
  Gain1 : Gain  Gain=1/(2*0.127)
  Scope : Scope  NumInputPorts=2
  Sqrt : Sqrt  SaturateOnIntegerOverflow=on
  Sqrt1 : Sqrt  SaturateOnIntegerOverflow=on
  Square : Math  Operator=square  SignedPower=off  SaturateOnIntegerOverflow=on
  Square1 : Math  Operator=square  SignedPower=off  SaturateOnIntegerOverflow=on
  Square2 : Math  Operator=square  SignedPower=off  SaturateOnIntegerOverflow=on
  Sum : Sum  Inputs=|+-
  Sum1 : Sum  Inputs=|++
  Sum2 : Sum  Inputs=|++
  Sum3 : Sum  Inputs=|+-
  Sum4 : Sum  Inputs=|+-
  theta_a1 : Outport
  theta_a2 : Outport  Port=2
  wires:
  Atan2/1 -> Scope/1, Sum3/1  "beta1"
  Sum2/1 -> Sqrt1/1
  Square1/1 -> Sum2/1, Sum1/2  "y^2"
  Acos/1 -> Sum3/2  "alpha1"
  Atan1/1 -> Scope/2, Sum4/1  "beta2"
  x/1 -> Atan2/2, Sum/1, Square/1  "x"
  Gain1/1 -> Acos/1
  Sum/1 -> Atan1/2, Square2/1  "x -2L"
  Gain/1 -> Acos1/1
  Acos1/1 -> Sum4/2  "alpha2"
  y/1 -> Atan1/1, Atan2/1, Square1/1  "y"
  Sum1/1 -> Sqrt/1
  Sqrt1/1 -> Gain/1  "d2"
  Square/1 -> Sum1/1  "x^2"
  Square2/1 -> Sum2/2  "(x -2L)^2"
  Constant1/1 -> Sum/2
  Sqrt/1 -> Gain1/1  "d1"
  Sum3/1 -> theta_a1/1  "theta_a1"
  Sum4/1 -> Bias/1  "theta_a2"
  Bias/1 -> theta_a2/1

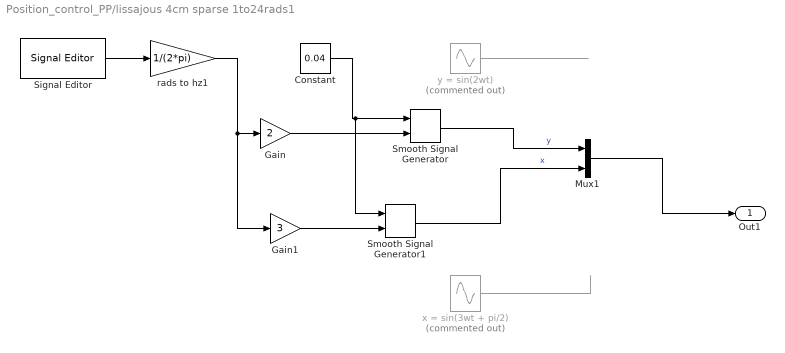
== system Position_control_PP/lissajous 4cm sparse 1to24rads1 ==
  Constant : Constant  Value=0.04
  Gain : Gain  Gain=2
  Gain1 : Gain  Gain=3
  Mux1 : Mux  Inputs=2
  Signal Editor : SignalEditorBlockLib/Signal Editor  FileName=lissajous_base_omega.mat  ActiveScenario=liisajous  ActiveSignal=ome  IsBus=off  OutputBusObjectStr=Bus: BusObject  SampleTime=0  Interpolate=off  ZeroCross=off  OutputAfterFinalValue=Setting to zero  Unit=inherit  PreserveSignalName=on
      settings: SourceProductName=Simulink
  Smooth Signal Generator : quarc_library/Sources/Signals/Smooth Signal Generator  signal_type=Sine  source=External (input ports)  amplitude=1  frequency=1  initial_phase=0  sample_time=qc_get_step_size  output_cos=off
      settings: SourceProductName=QUARC Targets
  Smooth Signal Generator1 : quarc_library/Sources/Signals/Smooth Signal Generator  signal_type=Sine  source=External (input ports)  amplitude=1  frequency=1  initial_phase=pi/2  sample_time=qc_get_step_size  output_cos=off
      settings: SourceProductName=QUARC Targets
  rads to hz1 : Gain  Gain=1/(2*pi)
  x = sin(3wt + pi/2) : Sin  Commented=on  Amplitude=0.04  Frequency=3  Phase=pi/2  SampleTime=0
  y = sin(2wt) : Sin  Commented=on  Amplitude=0.04  Frequency=2  SampleTime=0
  Out1 : Outport
  wires:
  y = sin(2wt)/1 -> ?
  x = sin(3wt + pi/2)/1 -> ?
  Mux1/1 -> Out1/1
  Constant/1 -> Smooth Signal Generator1/1, Smooth Signal Generator/1
  Signal Editor/1 -> rads to hz1/1
  rads to hz1/1 -> Gain1/1, Gain/1
  Gain/1 -> Smooth Signal Generator/2
  Gain1/1 -> Smooth Signal Generator1/2
  Smooth Signal Generator1/1 -> Mux1/2  "x"
  Smooth Signal Generator/1 -> Mux1/1  "y"

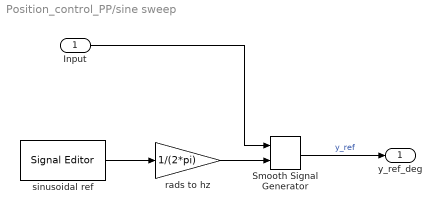
== system Position_control_PP/sine sweep ==
  Input : Inport
  Smooth Signal Generator : quarc_library/Sources/Signals/Smooth Signal Generator  signal_type=Sine  source=External (input ports)  amplitude=1  frequency=1  initial_phase=0  sample_time=qc_get_step_size  output_cos=off
      settings: SourceProductName=QUARC Targets
  rads to hz : Gain  Gain=1/(2*pi)
  sinusoidal ref : SignalEditorBlockLib/Signal Editor  FileName=angle_ref_scenario_freq.mat  ActiveScenario=x1to34_sparse  ActiveSignal=Signal 1  IsBus=off  OutputBusObjectStr=Bus: BusObject  SampleTime=0  Interpolate=off  ZeroCross=off  OutputAfterFinalValue=Holding final value  Unit=inherit  PreserveSignalName=on
      settings: SourceProductName=Simulink
  y_ref_deg : Outport
  wires:
  Input/1 -> Smooth Signal Generator/1
  sinusoidal ref/1 -> rads to hz/1
  rads to hz/1 -> Smooth Signal Generator/2
  Smooth Signal Generator/1 -> y_ref_deg/1  "y_ref"

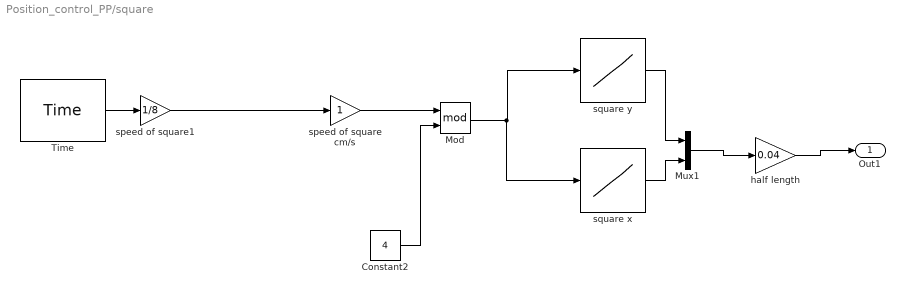
== system Position_control_PP/square ==
  Constant2 : Constant  Value=4
  Mod : Math  Operator=mod  SignedPower=off  SaturateOnIntegerOverflow=on
  Mux1 : Mux  Inputs=2
  Time : quarc_library/Sources/Time/Time  time_source=Wall clock  sample_time=qc_get_step_size
  half length : Gain  Gain=0.04
  speed of square cm/s : Gain
  speed of square1 : Gain  Gain=1/8
  square x : Lookup_n-D  NumberOfTableDimensions=1  BreakpointsForDimension1=0:4  Table=[-1, 1 , 1 , -1 ,-1]  InternalRulePriority=Speed  RndMeth=Simplest  InputSameDT=on
  square y : Lookup_n-D  NumberOfTableDimensions=1  BreakpointsForDimension1=0:4  Table=[-1, -1 , 1 , 1 ,-1]  InternalRulePriority=Speed  RndMeth=Simplest  InputSameDT=on
  Out1 : Outport
  wires:
  square y/1 -> Mux1/1
  Time/1 -> speed of square1/1
  Constant2/1 -> Mod/2
  Mux1/1 -> half length/1
  Mod/1 -> square y/1, square x/1
  square x/1 -> Mux1/2
  speed of square cm/s/1 -> Mod/1
  half length/1 -> Out1/1
  speed of square1/1 -> speed of square cm/s/1

== system Position_control_PP/untitledPanel ==
  Lamp1 : LampBlock  Tag=HiddenForWebPanel  PanelInfo="{\"panelId\":\"panelId-9ed59f3f-f720-46ec-8084-1779a040fe60\",\"type\":\"panelChild\",\"version\":\"2019b\",\"zIndex\":1500001}"
  panelInfo : PanelWebBlock  Tag=HiddenForWebPanel  PanelInfo="{\"compacted\":false,\"height\":115,\"left\":1684,\"panelId\":\"panelId-9ed59f3f-f720-46ec-8084-1779a040fe60\",\"top\":154,\"type\":\"panel\",\"version\":\"2019b\",\"visible\":true,\"width\":121,\"zIndex\":1500001}"

== system Position_control_PP/untitledPanel1 ==
  Lamp : LampBlock  Tag=HiddenForWebPanel  PanelInfo="{\"panelId\":\"panelId-49490bdd-6a45-4712-8d72-65ed97b81909\",\"type\":\"panelChild\",\"version\":\"2019b\",\"zIndex\":1500001}"
  panelInfo : PanelWebBlock  Tag=HiddenForWebPanel  PanelInfo="{\"compacted\":false,\"height\":115,\"left\":1685,\"panelId\":\"panelId-49490bdd-6a45-4712-8d72-65ed97b81909\",\"top\":32,\"type\":\"panel\",\"version\":\"2019b\",\"visible\":true,\"width\":121,\"zIndex\":1500002}"

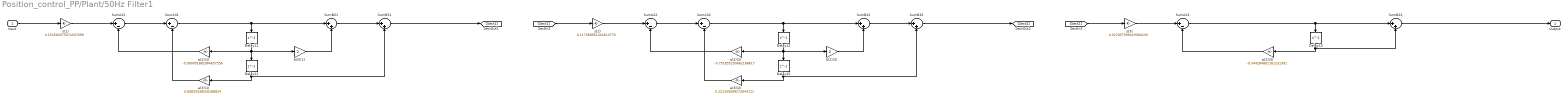
== system Position_control_PP/Plant/50Hz Filter1 ==
  Input : Inport
  Delay{11..13,21..22} (5 alike) : Delay  DelayLength=1  InitialCondition=0
  SumA{21..23,31..32} (5 alike) : Sum  Inputs=|+-  RndMeth=Nearest  SaturateOnIntegerOverflow=on  OutDataTypeStr=Inherit: Same as first input
  SumB{21..23,31..32} (5 alike) : Sum  Inputs=|++  RndMeth=Nearest  SaturateOnIntegerOverflow=on  OutDataTypeStr=Inherit: Same as first input
  a(2)(1) : Gain  Gain=-0.990091882984657556  ParamDataTypeStr=double  RndMeth=Nearest  SaturateOnIntegerOverflow=on  OutDataTypeStr=Inherit: Same as input
  a(2)(2) : Gain  Gain=-0.751855293662188617  ParamDataTypeStr=double  RndMeth=Nearest  SaturateOnIntegerOverflow=on  OutDataTypeStr=Inherit: Same as input
  a(2)(3) : Gain  Gain=-0.344284801161231391  ParamDataTypeStr=double  RndMeth=Nearest  SaturateOnIntegerOverflow=on  OutDataTypeStr=Inherit: Same as input
  a(3)(1) : Gain  Gain=0.60833338328188824  ParamDataTypeStr=double  RndMeth=Nearest  SaturateOnIntegerOverflow=on  OutDataTypeStr=Inherit: Same as input
  a(3)(2) : Gain  Gain=0.221335099272643721  ParamDataTypeStr=double  RndMeth=Nearest  SaturateOnIntegerOverflow=on  OutDataTypeStr=Inherit: Same as input
  b(2)(1) : Gain  Gain=2  ParamDataTypeStr=double  RndMeth=Nearest  SaturateOnIntegerOverflow=on  OutDataTypeStr=Inherit: Same as input
  b(2)(2) : Gain  Gain=2  ParamDataTypeStr=double  RndMeth=Nearest  SaturateOnIntegerOverflow=on  OutDataTypeStr=Inherit: Same as input
  s(1) : Gain  Gain=0.154560375074307699  ParamDataTypeStr=double  RndMeth=Nearest  SaturateOnIntegerOverflow=on  OutDataTypeStr=Inherit: Same as input
  s(2) : Gain  Gain=0.117369951402613776  ParamDataTypeStr=double  RndMeth=Nearest  SaturateOnIntegerOverflow=on  OutDataTypeStr=Inherit: Same as input
  s(3) : Gain  Gain=0.327857599419384249  ParamDataTypeStr=double  RndMeth=Nearest  SaturateOnIntegerOverflow=on  OutDataTypeStr=Inherit: Same as input
  Output : Outport
  wires:
  Input/1 -> s(1)/1
  s(1)/1 -> SumA21/1
  SumA21/1 -> SumA31/1
  SumA31/1 -> SumB21/1, Delay11/1
  SumB21/1 -> SumB31/1
  SumB31/1 -> [Sect1]
  a(2)(1)/1 -> SumA21/2
  Delay11/1 -> a(2)(1)/1, b(2)(1)/1, Delay21/1
  b(2)(1)/1 -> SumB21/2
  a(3)(1)/1 -> SumA31/2
  Delay21/1 -> a(3)(1)/1, SumB31/2
  [Sect1] -> s(2)/1
  s(2)/1 -> SumA22/1
  SumA22/1 -> SumA32/1
  SumA32/1 -> SumB22/1, Delay12/1
  SumB22/1 -> SumB32/1
  SumB32/1 -> [Sect2]
  a(2)(2)/1 -> SumA22/2
  Delay12/1 -> a(2)(2)/1, b(2)(2)/1, Delay22/1
  b(2)(2)/1 -> SumB22/2
  a(3)(2)/1 -> SumA32/2
  Delay22/1 -> a(3)(2)/1, SumB32/2
  [Sect2] -> s(3)/1
  s(3)/1 -> SumA23/1
  SumA23/1 -> SumB23/1, Delay13/1
  SumB23/1 -> Output/1
  a(2)(3)/1 -> SumA23/2
  Delay13/1 -> a(2)(3)/1, SumB23/2

== matlab function Position_control_PP/Plant/MATLAB Function1 ==
  data: u input; y output; upper_0 input; lower_0 input; upper_1 input; lower_1 input; bias input
function y = test_bounds(u, upper_0, lower_0, upper_1, lower_1,bias)
%#codegen
%  0 = everything ok
%  1 = low voltage
%  2 = shutting down
if bias
     upper_0 = upper_0 + pi/2;
     lower_0 = lower_0 + pi/2; 
     upper_1 = upper_1 + pi/2;
     lower_1 = lower_1 + pi/2;
end

if u<upper_0 && u>lower_0
    y = 0;
elseif u<upper_1 && u>lower_1
    y = 1;
else
    y = 2;
end

== matlab function Position_control_PP/Plant/MATLAB Function ==
  data: u input; y output; upper_0 input; lower_0 input; upper_1 input; lower_1 input
function y = test_bounds(u, upper_0, lower_0, upper_1, lower_1)
%#codegen
%  0 = everything ok
%  1 = low voltage
%  2 = shutting down
if u<upper_0 && u>lower_0
    y = 0;
elseif u<upper_1 && u>lower_1
    y = 1;
else
    y = 2;
end

== matlab function Position_control_PP/feed forward calculator ==
  data: t_a1 input; q1_dot output; t_a2 input; vx input; vy input; q2_dot output
function [q1_dot,q2_dot]  = ang_speed_ff(t_a1,t_a2,vx,vy)
%JACOBIAN_VF_PROJECTION Projection of v onto angle velocity
%   Detailed explanation goes here
alpha_dots = jacobian_vf_projection(t_a1,t_a2+pi/2,vx,vy);
q1_dot = alpha_dots(1);
q2_dot = alpha_dots(2);
end
